simulink subsystem "steps4harm"  (R2023b)
settings: Solver=VariableStepAuto  StartTime=0.0  StopTime=10.0  RelTol=1e-3
undefined symbols (not defined in the file): nHarmonics, shuntHarmonicsCorrected
settings Model: Creator=Veimar  LastModifiedBy=Veimar

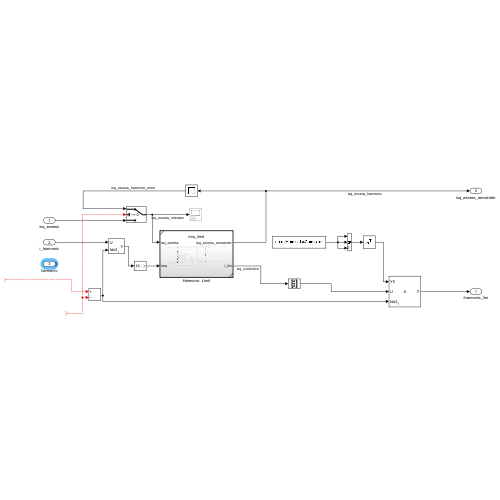
[thumbnail: Simulink's stored preview of the top-level diagram]
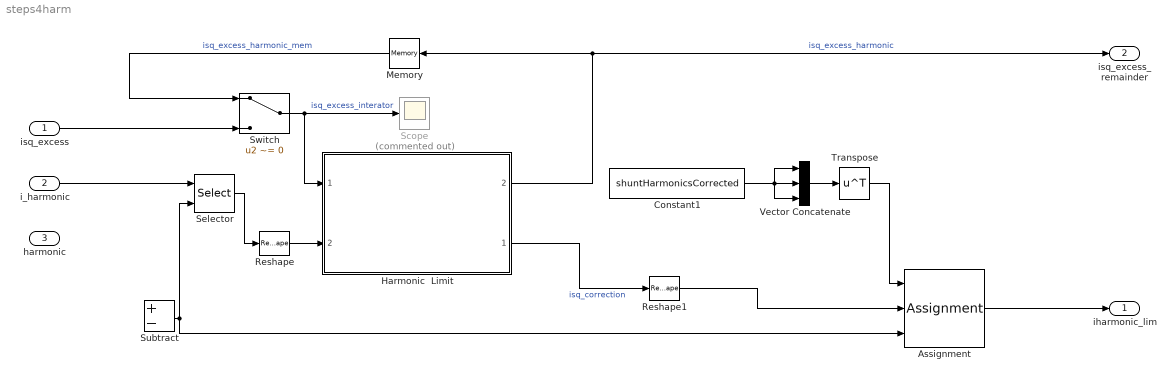
== system steps4harm ==
  isq_excess : Inport
  i_harmonic : Inport  Port=2
  harmonic : Inport  Port=3
  Assignment : Assignment  NumberOfDimensions=2  DiagnosticForDimensions=Warning  IndexOptions=Assign all,Index vector (port)  Indices=1,1  OutputSizes=3,nHarmonics
  Constant1 : Constant  Value=shuntHarmonicsCorrected  OutDataTypeStr=single
  Harmonic  Limit : Subsystem  TreatAsAtomicUnit=on  ReferencedSubsystem=rms_limit
      settings: PortSchema="{\"entries\":[{\"content\":{\"sides\":[{\"content\":{\"connectorIds\":[\"In1\",\"In2\"]},\"type\":\"ConnectorPlacement.EquallySpacedRectSide\",\"uuid\":\"a0edda42-1093-4dc5-a0fa-0d45baad0397\"},{\"content\":{\"connectorIds\":[\"Out2\",\"Out1\"],\"side\":\"RIGHT\"},\"type\":\"ConnectorPlacement.EquallySpacedRectSide\",\"uuid\":\"9461ca2c-2d49-476d-8dbf-46c4cd226d1a\"},{\"content\":{\"side\":\"TOP\"},\"type\":\"ConnectorPlacement.EquallySpacedRectSide\",\"uuid\":\"ebbd8734-3f86-4c2e-9126-3af595b2078a\"}]},\"type\":\"ConnectorPlacement.EquallySpacedConnector\",\"uuid\":\"3414606b-6b7d-4413-9cd8-bdd988f6d4a8\"}],\"packageUris\":[\"http://schema.mathworks.com/mf0/Connector/R2020b\"],\"version\":\"1.0\"}"
  Memory : Memory  InheritSampleTime=on
  Reshape : Reshape
  Reshape1 : Reshape  OutputDimensionality=Column vector (2-D)
  Scope : Scope  Commented=on
  Selector : Selector  NumberOfDimensions=2  InputPortWidth=1  IndexOptions=Select all,Index vector (port)  Indices=[1 3],1  OutputSizes=1,1
  Subtract : Sum  Inputs=+-
  Switch : Switch  Criteria=u2 ~= 0  Threshold=1  SaturateOnIntegerOverflow=off  InputSameDT=off
  Transpose : Math  Operator=transpose
  Vector Concatenate : Concatenate  NumInputs=3  Mode=Multidimensional array  ConcatenateDimension=2
  iharmonic_lim : Outport  OutDataTypeStr=single
  isq_excess_remainder : Outport  Port=2  OutDataTypeStr=single
  wires:
  Vector Concatenate/1 -> Transpose/1
  Transpose/1 -> Assignment/1
  isq_excess/1 -> Switch/3
  Constant1/1 -> Vector Concatenate/2, Vector Concatenate/1, Vector Concatenate/3
  i_harmonic/1 -> Selector/1
  Harmonic  Limit/2 -> Memory/1, isq_excess_remainder/1  "isq_excess_harmonic"
  Selector/1 -> Reshape/1
  Reshape/1 -> Harmonic  Limit/2
  Switch/1 -> Harmonic  Limit/1, Scope/1  "isq_excess_interator"
  Reshape1/1 -> Assignment/2
  Subtract/1 -> Selector/2, Assignment/3
  Harmonic  Limit/1 -> Reshape1/1  "isq_correction"
  Memory/1 -> Switch/1  "isq_excess_harmonic_mem"
  ? -> Switch/2, Subtract/2
  Assignment/1 -> iharmonic_lim/1
  ? -> Subtract/1
